simulink subsystem "deser222"  (R2024a)
settings: Solver=VariableStepAuto  StartTime=0.0  StopTime=10.0  RelTol=1e-3
model mask{edge_triggered=off}
  mask prompts: edge_triggered "Data enable is edge triggered."
InitFcn:
  | %% DSPBuilder Start
  | alt_dspbuilder_update_model(bdroot)
  | %% DSPBuilder End
StartFcn:
  | %% DSPBuilder Start
  | alt_dspbuilder_hdlimport_prepare_for_simulation(bdroot)
  | %% DSPBuilder End
libraries: allblocks_alteradspbuilder2 x10
settings Model: Creator=vboxuser  LastModifiedBy=piotr
settings SolverCC: AlgebraicLoopSolver=TrustRegion
settings DebuggingCC: UnconnectedInputMsg=warning  UnconnectedOutputMsg=warning  UnconnectedLineMsg=warning
settings ModelReferenceCC: EnableRefExpFcnMdlSchedulingChecks=on
settings RTWCC: GPUComputeCapability=3.5

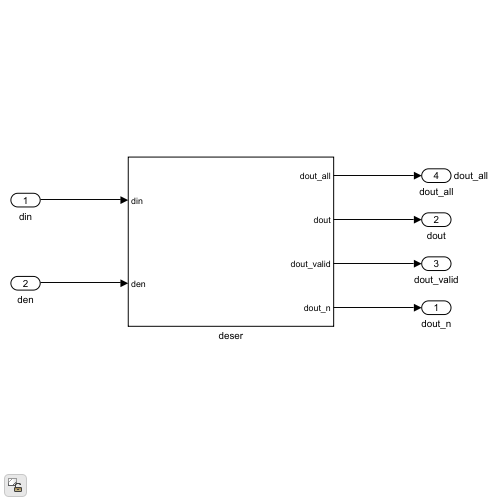
[thumbnail: Simulink's stored preview of the top-level diagram]
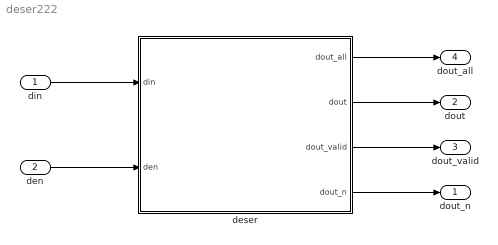
== system deser222 ==
  din : Inport
  den : Inport  Port=2
  deser : Subsystem
  dout_n : Outport
  dout : Outport  Port=2
  dout_valid : Outport  Port=3
  dout_all : Outport  Port=4  SignalName=dout_all
  wires:
  din/1 -> deser/1(din)
  den/1 -> deser/2(den)
  deser/2(dout) -> dout/1
  deser/1(dout_all) -> dout_all/1
  deser/4(dout_n) -> dout_n/1
  deser/3(dout_valid) -> dout_valid/1

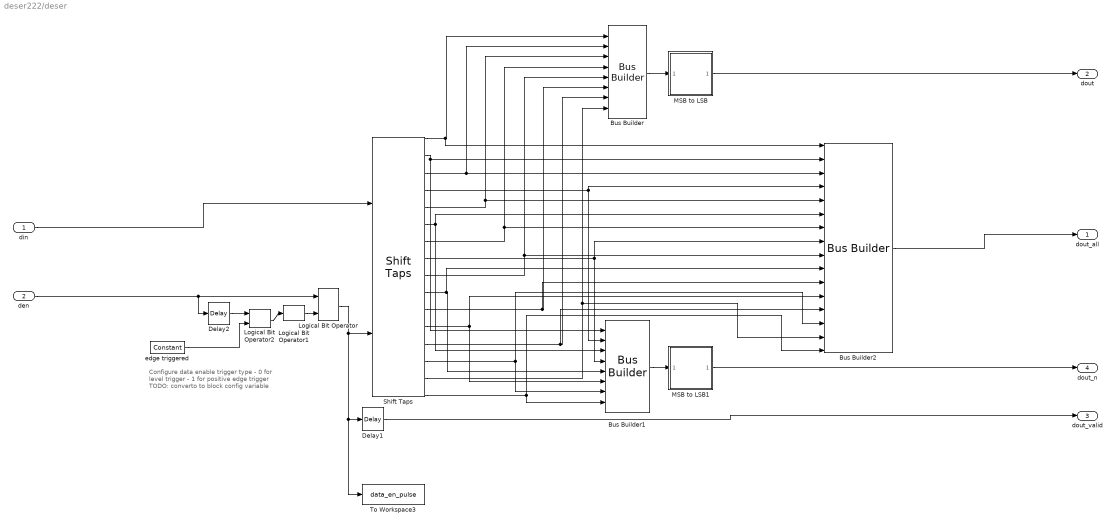
== system deser222/deser ==
  note: Configure data enable trigger type
      |  - 0 for level trigger
      |  - 1 for positive edge trigger
      |
      | TODO: converto to block config variable
  din : Inport
  den : Inport  Port=2
  Bus Builder : allblocks_alteradspbuilder2/Bus Builder  BusType=Unsigned Integer  bwl=8  bwr=1  pipeline_display=0
  Bus Builder1 : allblocks_alteradspbuilder2/Bus Builder  BusType=Unsigned Integer  bwl=8  bwr=1  pipeline_display=0
  Bus Builder2 : allblocks_alteradspbuilder2/Bus Builder  BusType=Unsigned Integer  bwl=16  bwr=1  pipeline_display=0
  Delay1 : allblocks_alteradspbuilder2/Delay  pipeline=1  pipeline_display=1  ClockPhase=1  use_ena=off  use_sclr=off  allowFloatingPointOverride=on  logOutputs=off  logFile=D:\programowanie\studia\ids\system2\tb_deser\deser_deser_Delay1.fixedpointlog  use_init=off  reset_value=1
  Delay2 : allblocks_alteradspbuilder2/Delay  pipeline=1  pipeline_display=1  ClockPhase=1  use_ena=off  use_sclr=off  allowFloatingPointOverride=on  logOutputs=off  logFile=D:\programowanie\studia\ids\system2\tb_deser\deser_deser_Delay2.fixedpointlog  use_init=off  reset_value=1
  Logical Bit Operator : allblocks_alteradspbuilder2/Logical Bit Operator  LogicalOperator=AND  user_inputs=2  pipeline_display=0
  Logical Bit Operator1 : allblocks_alteradspbuilder2/Logical Bit Operator  LogicalOperator=NOT  user_inputs=2  pipeline_display=0
  Logical Bit Operator2 : allblocks_alteradspbuilder2/Logical Bit Operator  LogicalOperator=AND  user_inputs=2  pipeline_display=0
  MSB to LSB : Subsystem  ReferencedSubsystem=MSB_to_LSB
  MSB to LSB1 : Subsystem  ReferencedSubsystem=MSB_to_LSB
  Shift Taps : allblocks_alteradspbuilder2/Shift Taps  number_of_taps=16  tap_distance=sym_samples  use_shiftout=off  use_ena=on  use_sclr=off  use_dedicated_circuitry=on  ram_type=AUTO  allowFloatingPointOverride=on  logOutputs=off  logFile=D:\programowanie\studia\ids\system2\tb_deser\deser_deser_Shift+Taps%3A%3At.fixedpointlog,D:\programowanie\studia\ids\system2\tb_deser\deser_deser_Shift+Taps%3A%3At.fixedpointlog,D:\programowanie\studia\ids\system2\tb_deser\deser_deser_Shift+Taps%3A%3At.fixedpointlog,D:\programowanie\studia\ids\system2\tb_deser\deser_deser_Shift+Taps%3A%3At.fixedpointlog,D:\programowanie\studia\ids\system2\tb_deser\deser_deser_Shift+Taps%3A%3At.fixedpointlog,D:\programowanie\studia\ids\system2\tb_deser\deser_deser_Shift+Taps%3A%3At.fixedpointlog,D:\programowanie\studia\ids\system2\tb_deser\deser_deser_Shift+Taps%3A%3At.fixedpointlog,D:\programowanie\studia\ids\system2\tb_deser\deser_deser_Shift+Taps%3A%3At.fixedpointlog,D:\programowanie\studia\ids\system2\tb_deser\deser_deser_Shift+Taps%3A%3At.fixedpointlog,D:\programowanie\studia\ids\system2\tb_deser\deser_deser_Shift+Taps%3A%3At.fixedpointlog,D:\programowanie\studia\ids\system2\tb_deser\deser_deser_Shift+Taps%3A%3At.fixedpointlog,D:\programowanie\studia\ids\system2\tb_deser\deser_deser_Shift+Taps%3A%3At.fixedpointlog,D:\programowanie\studia\ids\system2\tb_deser\deser_deser_Shift+Taps%3A%3At.fixedpointlog,D:\programowanie\studia\ids\system2\tb_deser\deser_deser_Shift+Taps%3A%3At.fixedpointlog,D:\programowanie\studia\ids\system2\tb_deser\deser_deser_Shift+Taps%3A%3At.fixedpointlog,D:\programowanie\studia\ids\system2\tb_deser\deser_deser_Shift+Taps%3A%3At.fixedpointlog,
  To Workspace3 : ToWorkspace  VariableName=data_en_pulse  SampleTime=-1
      settings: Save2DSignal=2-D array (concatenate along first dimension)
  edge triggered : allblocks_alteradspbuilder2/Constant  mask_cst=edge_triggered  BusType=Single Bit  bwl=8  bwr=0  roundMode=Truncate  satMode=Wrap  SpecifyClock=off  allowFloatingPointOverride=on  logOutputs=off  logFile=D:\programowanie\studia\ids\system2\tb_deser\deser_deser_edge+triggered.fixedpointlog
  dout_all : Outport
  dout : Outport  Port=2
  dout_valid : Outport  Port=3
  dout_n : Outport  Port=4
  wires:
  Shift Taps/6 -> Bus Builder2/6, Bus Builder1/3
  Shift Taps/5 -> Bus Builder/3, Bus Builder2/5
  Bus Builder/1 -> MSB to LSB/1
  Shift Taps/2 -> Bus Builder1/1, Bus Builder2/2
  Shift Taps/3 -> Bus Builder2/3, Bus Builder/2
  Delay2/1 -> Logical Bit Operator2/1
  Shift Taps/4 -> Bus Builder2/4, Bus Builder1/2
  Shift Taps/16 -> Bus Builder1/8, Bus Builder2/16
  Shift Taps/11 -> Bus Builder2/11, Bus Builder/6
  Bus Builder1/1 -> MSB to LSB1/1
  Shift Taps/15 -> Bus Builder/8, Bus Builder2/15
  Shift Taps/9 -> Bus Builder2/9, Bus Builder/5
  Shift Taps/13 -> Bus Builder2/13, Bus Builder/7
  Logical Bit Operator2/1 -> Logical Bit Operator1/1
  Bus Builder2/1 -> dout_all/1
  Shift Taps/1 -> Bus Builder2/1, Bus Builder/1
  Delay1/1 -> dout_valid/1
  Shift Taps/14 -> Bus Builder1/7, Bus Builder2/14
  Shift Taps/10 -> Bus Builder2/10, Bus Builder1/5
  Logical Bit Operator/1 -> Delay1/1, To Workspace3/1, Shift Taps/2
  Shift Taps/7 -> Bus Builder/4, Bus Builder2/7
  Shift Taps/12 -> Bus Builder2/12, Bus Builder1/6
  Logical Bit Operator1/1 -> Logical Bit Operator/2
  den/1 -> Delay2/1, Logical Bit Operator/1
  Shift Taps/8 -> Bus Builder1/4, Bus Builder2/8
  MSB to LSB1/1 -> dout_n/1
  edge triggered/1 -> Logical Bit Operator2/2
  MSB to LSB/1 -> dout/1
  din/1 -> Shift Taps/1
